simulink model "polagacy"  (R2019a)
settings: Solver=VariableStepAuto  StartTime=0.0  StopTime=20  RelTol=1e-3
values from neighbouring files (symbols this model uses):
  T = 2e-3    (= 0.002)    [poxi_raws.m]
undefined symbols (not defined in the file or in its folder): A_buhp, A_bulp, B_buhp, B_bulp
settings Model: Creator=Admin  LastModifiedBy=Admin

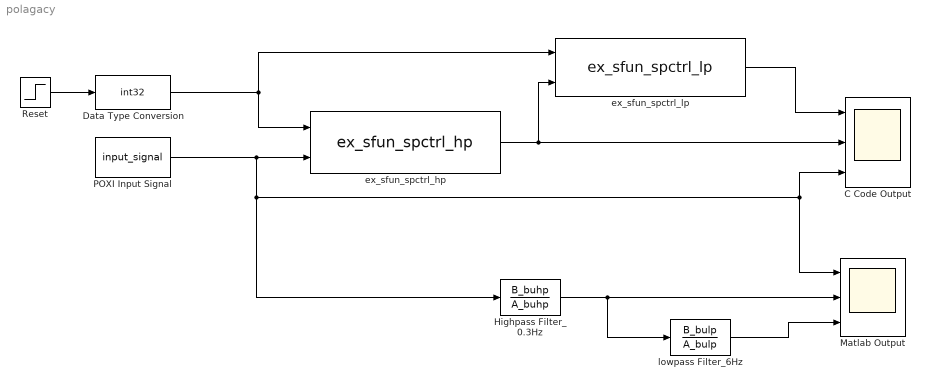
== system polagacy ==
  C Code Output : Scope  NumInputPorts=3
  Data Type Conversion : DataTypeConversion  OutDataTypeStr=int32
  Highpass Filter_0.3Hz : DiscreteTransferFcn  Numerator=B_buhp  Denominator=A_buhp
  Matlab Output : Scope  NumInputPorts=3
  POXI Input Signal : FromWorkspace  VariableName=input_signal  OutDataTypeStr=double  SampleTime=T
  Reset : Step  Time=0.001  Before=1  After=0  SampleTime=0
  ex_sfun_spctrl_hp : S-Function  FunctionName=ex_sfun_spctrl_hp  SFunctionDeploymentMode=off  EnableBusSupport=off  mask(Legacy Function){SFunctionSpec=double y1 = pofilt_hp(int32 u1, double u2), ShowSpec=on}
      mask prompts: ShowSpec "Display function specification"
      mask help:
      | This block allows you to call the legacy functions specified by the following Legacy Code Tool definition:
      | def.SFunctionName = 'ex_sfun_spctrl_hp';
      | def.OutputFcnSpec = 'double y1 = pofilt_hp(int32 u1, double u2)';
      | def.HeaderFiles = {'pofilt_hp.h'};
      mask Help: <p>This block was generated automatically by the Legacy Code Tool. For detailed help on this tool, call<a href="matlab:legacy_code('help')"> legacy_code('help')</a>.</p>
      mask Callback ShowSpec:
      | if strcmp(get_param(gcbh, 'ShowSpec'), 'on')
      |   set_param(gcbh, 'MaskDisplay', sprintf('fprintf(''%s'');', get_param(gcbh, 'SFunctionSpec')));
      | else
      |   set_param(gcbh, 'MaskDisplay', sprintf('fprintf(''%s'');', get_param(gcbh, 'FunctionName')));
      | end
      mask Display: fprintf('double y1 = pofilt_hp(int32 u1, double u2)');
  ex_sfun_spctrl_lp : S-Function  FunctionName=ex_sfun_spctrl_lp  SFunctionDeploymentMode=off  EnableBusSupport=off  mask(Legacy Function){SFunctionSpec=double y1 = pofilt_lp(int32 u1, double u2), ShowSpec=on}
      mask prompts: ShowSpec "Display function specification"
      mask help:
      | This block allows you to call the legacy functions specified by the following Legacy Code Tool definition:
      | def.SFunctionName = 'ex_sfun_spctrl_lp';
      | def.OutputFcnSpec = 'double y1 = pofilt_lp(int32 u1, double u2)';
      | def.HeaderFiles = {'pofilt_lp.h'};
      mask Help: <p>This block was generated automatically by the Legacy Code Tool. For detailed help on this tool, call<a href="matlab:legacy_code('help')"> legacy_code('help')</a>.</p>
      mask Callback ShowSpec:
      | if strcmp(get_param(gcbh, 'ShowSpec'), 'on')
      |   set_param(gcbh, 'MaskDisplay', sprintf('fprintf(''%s'');', get_param(gcbh, 'SFunctionSpec')));
      | else
      |   set_param(gcbh, 'MaskDisplay', sprintf('fprintf(''%s'');', get_param(gcbh, 'FunctionName')));
      | end
      mask Display: fprintf('double y1 = pofilt_lp(int32 u1, double u2)');
  lowpass Filter_6Hz : DiscreteTransferFcn  Numerator=B_bulp  Denominator=A_bulp
  wires:
  POXI Input Signal/1 -> ex_sfun_spctrl_hp/2, Highpass Filter_0.3Hz/1, Matlab Output/1, C Code Output/3
  Reset/1 -> Data Type Conversion/1
  Data Type Conversion/1 -> ex_sfun_spctrl_lp/1, ex_sfun_spctrl_hp/1
  Highpass Filter_0.3Hz/1 -> lowpass Filter_6Hz/1, Matlab Output/2
  lowpass Filter_6Hz/1 -> Matlab Output/3
  ex_sfun_spctrl_hp/1 -> ex_sfun_spctrl_lp/2, C Code Output/2
  ex_sfun_spctrl_lp/1 -> C Code Output/1
